simulink model "AOO"  (R2022b)
settings: Solver=FixedStepAuto  StartTime=0.0  StopTime=10.0  FixedStep=1e-3  RelTol=1e-3  EnableMultiTasking=on
undefined symbols (not defined in the file): D10, D11, D12, D2, D5, D8, D9, PTA0, PTA2, PTB9, PTC4, PTD0, PTD2, PTD3
libraries: frdmk64flib x7
settings Model: ExtModeTrigDuration=5  Creator=Ali Umar  LastModifiedBy=seankhaira
settings OptimizationCC: EnhancedBackFolding=on  PassReuseOutputArgsAs=Individual arguments  ZeroExternalMemoryAtStartup=off  ZeroInternalMemoryAtStartup=off  MaxStackSize=64  OptimizeBlockOrder=speed  DifferentSizesBufferReuse=on  OptimizationCustomize=off  EfficientTunableParamExpr=on
settings DebuggingCC: ParameterTunabilityLossMsg=error
settings HardwareCC: ProdBitPerPointer=32  ProdBitPerSizeT=32  ProdBitPerPtrDiffT=32  ProdLargestAtomicInteger=Long  ProdLargestAtomicFloat=Double  ProdWordSize=32  ProdHWDeviceType=ARM Compatible->ARM Cortex
settings SFSimCC: MATLABDynamicMemAlloc=off
settings RTWCC: Description=Embedded Coder  SystemTargetFile=ert.tlc  HardwareBoard=NXP FRDM-K64F  TLCOptions="-aInlineSetEventsForThisBaseRateFcn=TLC_FALSE -aSuppressMultiTaskScheduler=TLC_FALSE  -aRateBasedStepFcn=0"  TemplateMakefile=ert_default_tmf  Toolchain=GNU Tools for ARM Embedded Processors
settings CodeAppCC: ForceParamTrailComments=on  IgnoreCustomStorageClasses=off  OperatorAnnotations=on  SimulinkDataObjDesc=on  SFDataObjDesc=on  InsertBlockDesc=on
settings ERTTargetCC: ExtModeTransport=4  ExtModeMexFile=sendToCommService

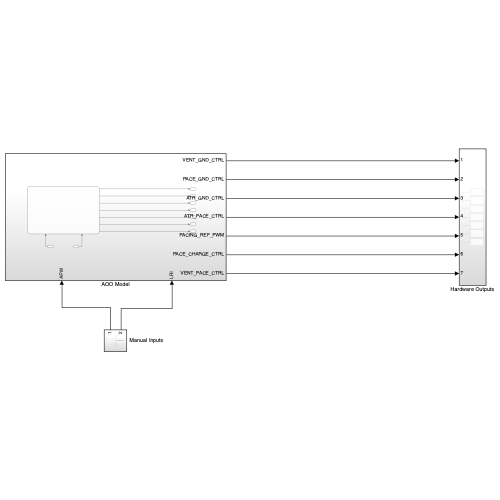
[thumbnail: Simulink's stored preview of the top-level diagram]
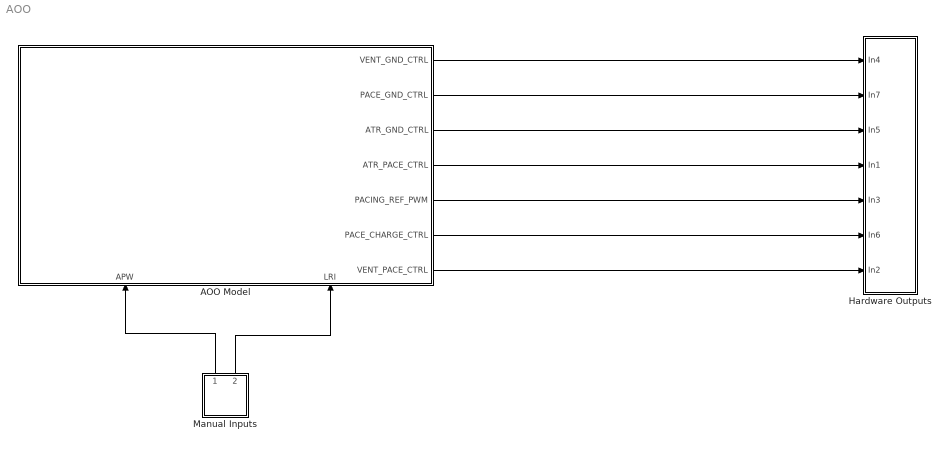
== system AOO ==
  AOO Model : Subsystem
      settings: PortSchema="{\"entries\":[{\"content\":{\"sides\":[{\"content\":{\"connectorIds\":[]},\"type\":\"ConnectorPlacement.EquallySpacedRectSide\",\"uuid\":\"51f6e257-d984-42e6-a2e1-3eb35c33020a\"},{\"content\":{\"connectorIds\":[\"Out1\",\"Out2\",\"Out3\",\"Out4\",\"Out5\",\"Out6\",\"Out7\"],\"side\":\"RIGHT\"},\"type\":\"ConnectorPlacement.EquallySpacedRectSide\",\"uuid\":\"15d7ca2c-4088-4eba-b8d1-9775bc9ae5f1\"},{\"content\":{\"connectorIds\":[],\"side\":\"TOP\"},\"type\":\"ConnectorPlacement.EquallySpacedRectSide\",\"uuid\":\"94f4e96f-03fb-4c15-8306-4cffcbe47276\"},{\"content\":{\"connectorIds\":[\"In1\",\"In2\"],\"side\":\"BOTTOM\"},\"type\":\"ConnectorPlacement.EquallySpacedRectSide\",\"uuid\":\"5f11c2eb-0470-4a15-953e-07a0d0e4eb63\"}]},\"type\":\"ConnectorPlacement.EquallySpacedConnector\",\"uuid\":\"61b376fb-6cc0-4d98-8932-bb572b9f6268\"}],\"packageUris\":[\"http://schema.mathworks.com/mf0/Connector/R2020b\"],\"version\":\"1.0\"}"
  Hardware Outputs : Subsystem
  Manual Inputs : Subsystem
  wires:
  Manual Inputs/1(Out1) -> AOO Model/1(APW)
  Manual Inputs/2(Out2) -> AOO Model/2(LRI)
  AOO Model/1(VENT_GND_CTRL) -> Hardware Outputs/1(In4)
  AOO Model/2(PACE_GND_CTRL) -> Hardware Outputs/2(In7)
  AOO Model/3(ATR_GND_CTRL) -> Hardware Outputs/3(In5)
  AOO Model/4(ATR_PACE_CTRL) -> Hardware Outputs/4(In1)
  AOO Model/5(PACING_REF_PWM) -> Hardware Outputs/5(In3)
  AOO Model/6(PACE_CHARGE_CTRL) -> Hardware Outputs/6(In6)
  AOO Model/7(VENT_PACE_CTRL) -> Hardware Outputs/7(In2)

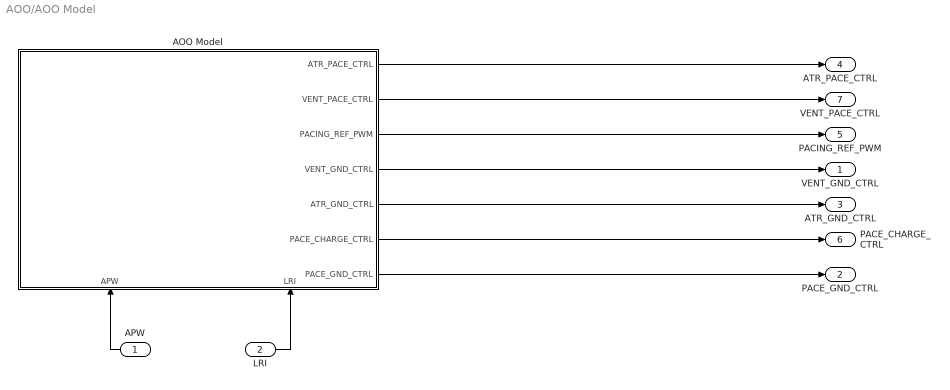
== system AOO/AOO Model ==
  APW : Inport
  LRI : Inport  Port=2
  AOO Model : Stateflow chart  TreatAsAtomicUnit=on
      settings: PortSchema="{\"entries\":[{\"content\":{\"sides\":[{\"content\":{\"connectorIds\":[]},\"type\":\"ConnectorPlacement.EquallySpacedRectSide\",\"uuid\":\"449a674f-8160-48ea-9d0e-c1dc2fe71515\"},{\"content\":{\"connectorIds\":[\"Out4\",\"Out7\",\"Out5\",\"Out1\",\"Out3\",\"Out6\",\"Out2\"],\"side\":\"RIGHT\"},\"type\":\"ConnectorPlacement.EquallySpacedRectSide\",\"uuid\":\"35702679-254d-49fa-8b13-2e5929d79215\"},{\"content\":{\"connectorIds\":[],\"side\":\"TOP\"},\"type\":\"ConnectorPlacement.EquallySpacedRectSide\",\"uuid\":\"818609a3-e142-415a-8096-b9af067f1b99\"},{\"content\":{\"connectorIds\":[\"In1\",\"In2\"],\"side\":\"BOTTOM\"},\"type\":\"ConnectorPlacement.EquallySpacedRectSide\",\"uuid\":\"0ccfb058-af85-432f-abdb-5391aedaf195\"}]},\"type\":\"ConnectorPlacement.EquallySpacedConnector\",\"uuid\":\"c932a4ac-b13d-4eda-80a2-7a8a0f724622\"}],\"packageUris\":[\"http://schema.mathworks.com/mf0/Connector/R2020b\"],\"version\":\"1.0\"}"
  VENT_GND_CTRL : Outport
  PACE_GND_CTRL : Outport  Port=2
  ATR_GND_CTRL : Outport  Port=3
  ATR_PACE_CTRL : Outport  Port=4
  PACING_REF_PWM : Outport  Port=5
  PACE_CHARGE_CTRL : Outport  Port=6
  VENT_PACE_CTRL : Outport  Port=7
  wires:
  AOO Model/4(ATR_PACE_CTRL) -> ATR_PACE_CTRL/1
  AOO Model/2(PACE_GND_CTRL) -> PACE_GND_CTRL/1
  AOO Model/3(ATR_GND_CTRL) -> ATR_GND_CTRL/1
  APW/1 -> AOO Model/1(APW)
  AOO Model/7(VENT_PACE_CTRL) -> VENT_PACE_CTRL/1
  AOO Model/1(VENT_GND_CTRL) -> VENT_GND_CTRL/1
  LRI/1 -> AOO Model/2(LRI)
  AOO Model/5(PACING_REF_PWM) -> PACING_REF_PWM/1
  AOO Model/6(PACE_CHARGE_CTRL) -> PACE_CHARGE_CTRL/1

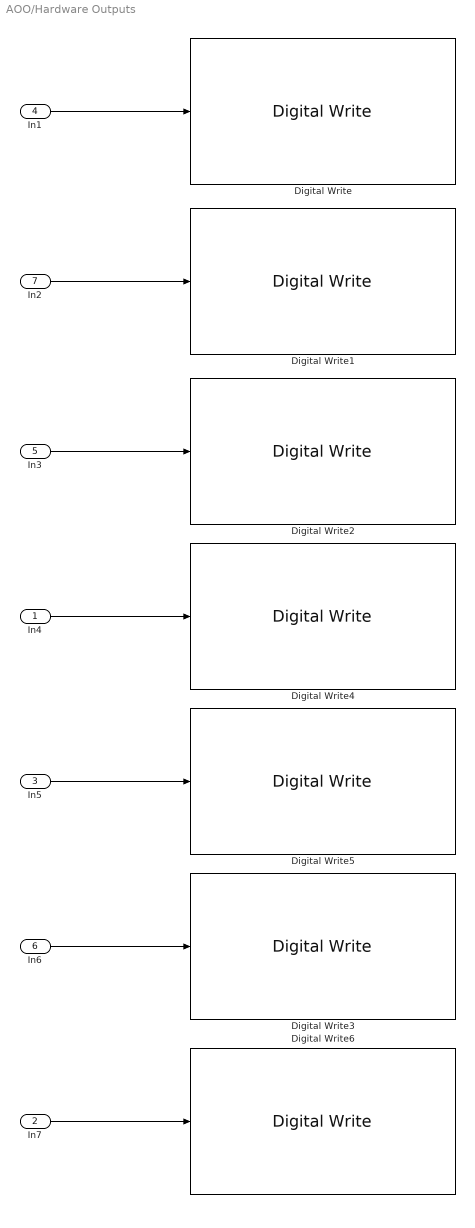
== system AOO/Hardware Outputs ==
  In4 : Inport
  In7 : Inport  Port=2
  In5 : Inport  Port=3
  In1 : Inport  Port=4
  In3 : Inport  Port=5
  In6 : Inport  Port=6
  In2 : Inport  Port=7
  Digital Write : frdmk64flib/Digital Write  Whichpin=PTA0 (D8)
  Digital Write1 : frdmk64flib/Digital Write  Whichpin=PTC4 (D9)
  Digital Write2 : frdmk64flib/Digital Write  Whichpin=PTA2 (D5)
  Digital Write3 : frdmk64flib/Digital Write  Whichpin=PTB9 (D2)
  Digital Write4 : frdmk64flib/Digital Write  Whichpin=PTD3 (D12)
  Digital Write5 : frdmk64flib/Digital Write  Whichpin=PTD2 (D11)
  Digital Write6 : frdmk64flib/Digital Write  Whichpin=PTD0 (D10)
  wires:
  In1/1 -> Digital Write/1
  In5/1 -> Digital Write5/1
  In3/1 -> Digital Write2/1
  In6/1 -> Digital Write3/1
  In7/1 -> Digital Write6/1
  In2/1 -> Digital Write1/1
  In4/1 -> Digital Write4/1

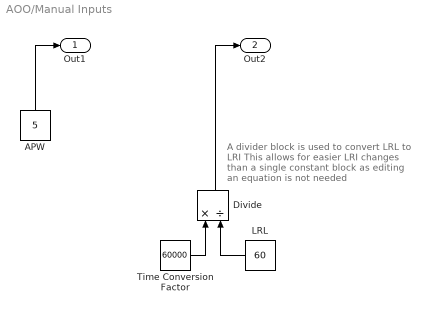
== system AOO/Manual Inputs ==
  note: A divider block is used to convert LRL to LRI
      | This allows for easier LRI changes than a single constant block as editing an equation is not needed
  APW : Constant  Value=5
  Divide : Product  Inputs=*/
  LRL : Constant  Value=60
  Time Conversion Factor : Constant  Value=60000
  Out1 : Outport
  Out2 : Outport  Port=2
  wires:
  Time Conversion Factor/1 -> Divide/1
  LRL/1 -> Divide/2
  Divide/1 -> Out2/1
  APW/1 -> Out1/1

== stateflow chart AOO/AOO Model/AOO Model ==
  state Charging_C22_Discharging_C21
    entry:
    %Charging C22
    ATR_PACE_CTRL = false;
    VENT_PACE_CTRL = false;
    PACING_REF_PWM  = 75;
    PACE_CHARGE_CTRL = true;
    %Discharging Backwards Capacitor
    PACE_GND_CTRL = true;
    VENT_PACE_CTRL = false;
    ATR_PACE_CTRL = false;
    VENT_GND_CTRL = false;
    ATR_GND_CTRL = true;
  note: Come back to charging state after pulse of APW length, so wait LRI - APW before next pulse
  state AOO_Pacing
    entry:
    PACE_CHARGE_CTRL = false;
    PACE_GND_CTRL = true;
    VENT_PACE_CTRL = false;
    ATR_GND_CTRL = false;
    VENT_GND_CTRL = false;
    ATR_PACE_CTRL = true;
  note: Pacing state discharges the pacing capacitor for an APW amount of time
  (default) -> Charging_C22_Discharging_C21
  Charging_C22_Discharging_C21 -> AOO_Pacing : after(LRI-APW,msec)
  AOO_Pacing -> Charging_C22_Discharging_C21 : after(APW,msec)
  data: VENT_GND_CTRL output; PACE_GND_CTRL output; ATR_GND_CTRL output; ATR_PACE_CTRL output; PACING_REF_PWM output; PACE_CHARGE_CTRL output; VENT_PACE_CTRL output; APW input; LRI input
